simulink library "ncukit"  (R2023b)
settings: Solver=VariableStepAuto  StartTime=0.0  StopTime=10.0  RelTol=1e-3
libraries: simulink x1
settings Model: Creator=sebam  LastModifiedBy=seb
settings SFSimCC: SimUserIncludeDirs=..\lib
settings SFSimCC: SimCustomHeaderCode=|
  | #include <gpio/gpio.h>
  | #include <can/can.h>
settings SFSimCC: SimUserSources=|
  | ..\lib\gpio\gpio.c
  | ..\lib\can\can.c
settings RTWCC: RTWUseSimCustomCode=on  CustomInclude=..\lib
settings RTWCC: CustomHeaderCode=|
  | #include <gpio/gpio.h>
  | #include <can/can.h>
settings RTWCC: CustomSource=|
  | ..\lib\gpio\gpio.c
  | ..\lib\can\can.c

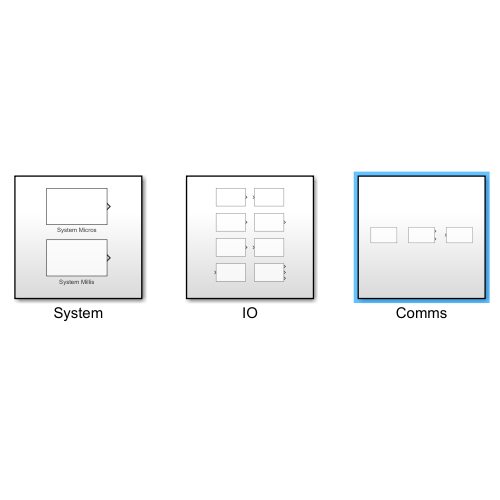
[thumbnail: Simulink's stored preview of the top-level diagram]
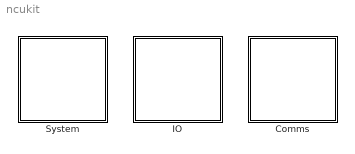
== system ncukit ==
  Comms : Subsystem
  IO : Subsystem
  System : Subsystem

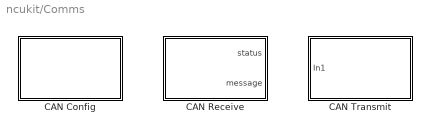
== system ncukit/Comms ==
  CAN Config : Subsystem  mask{bus=can_bus.CAN0, bitrate=can_bitrate.CAN_BITRATE_125K}
      mask Display: image('can_config.png', [25,7,50,50]);
  CAN Receive : Subsystem  mask{bus=can_bus.CAN0}
      mask Display: image('can_receive.png', [25,7,50,50]);
  CAN Transmit : Subsystem  mask{bus=can_bus.CAN0}
      mask Display: image('can_transmit.png', [25,7,50,50]);

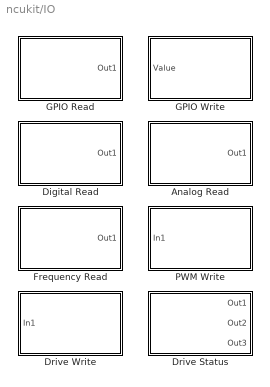
== system ncukit/IO ==
  Analog Read : Subsystem
      mask Display: image('analog_read.png', [25,7,50,50]);
  Digital Read : Subsystem
      mask Display: image('digital_read.png', [25,7,50,50]);
  Drive Status : Subsystem
      mask Display: image('drive_status.png', [25,7,50,50]);
  Drive Write : Subsystem
      mask Display: image('drive_write.png', [25,7,50,50]);
  Frequency Read : Subsystem
      mask Display: image('freq_read.png', [25,7,50,50]);
  GPIO Read : Subsystem  mask{pin=gpio_pin.LED1}
      mask Display: image('gpio_read.png', [25,7,50,50]);
  GPIO Write : Subsystem  mask{pin=gpio_pin.GPIO0}
      mask Display: image('gpio_write.png', [25,7,50,50]);
  PWM Write : Subsystem
      mask Display: image('pwm_write.png', [25,7,50,50]);

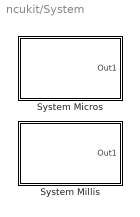
== system ncukit/System ==
  System Micros : Subsystem
      mask Display: image('system_us.png', [25,7,50,50]);
  System Millis : Subsystem
      mask Display: image('system_ms.png', [25,7,50,50]);

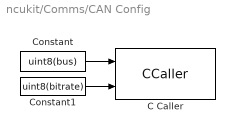
== system ncukit/Comms/CAN Config ==
  C Caller : CCaller  FunctionName=can_set_bitrate  PortSpecificationStruct="%)30     .    V ,   8    (     @         %    \"     (    !     0         %  0 \"0    $    _    07)G3F%M90  4&]R=$YA;64 4V-O<&4     26YD97@     5'EP90      4VEZ90      27-';&]B86P   X    P    !@    @    $          4    (     0    ,    !         !   P!B=7, #@   #     &    \"     0         !0    @    !     P    $         $  # &)U<P .    .     8    (    !          %    \"     $    %     0         0    !0   $EN<'5T    #@   #@    &    \"     8         !0    @    !     0    $         \"0    @               X    X    !@    @    $          4    (     0    4    !         !     %    =6EN=#@    .    ,     8    (    !          %    \"     $    !     0         0  $ ,0    X    P    !@    @    ) @        4    (     0    $    !          (  0      #@   #@    &    \"     0         !0    @    !    !P    $         $     <   !B:71R871E  X    X    !@    @    $          4    (     0    <    !         !     '    8FET<F%T90 .    .     8    (    !          %    \"     $    %     0         0    !0   $EN<'5T    #@   #@    &    \"     8         !0    @    !     0    $         \"0    @           #P/PX   !(    !@    @    $          4    (     0   !,    !         !     3    16YU;3H@8V%N7V)I=')A=&5?=       #@   #     &    \"     0         !0    @    !     0    $         $  ! #$    .    ,     8    (    \"0(        %    \"     $    !     0         \"  $"
  Constant : Constant  Value=uint8(bus)
  Constant1 : Constant  Value=uint8(bitrate)
  wires:
  Constant/1 -> C Caller/1
  Constant1/1 -> C Caller/2

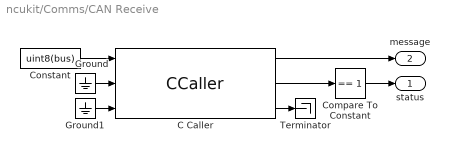
== system ncukit/Comms/CAN Receive ==
  C Caller : CCaller  FunctionName=can_receive  PortSpecificationStruct="%)30     .    . <   8    (     @         %    \"     0    !     0         %  0 \"0    $    _    07)G3F%M90  4&]R=$YA;64 4V-O<&4     26YD97@     5'EP90      4VEZ90      27-';&]B86P   X    P    !@    @    $          4    (     0    ,    !         !   P!O=70 #@   #     &    \"     0         !0    @    !     P    $         $  # &]U=  .    .     8    (    !          %    \"     $    &     0         0   ...(+2112 chars)"
  Compare To Constant : simulink/Logic and Bit Operations/Compare To Constant  relop===  const=1  OutDataTypeStr=boolean
  Constant : Constant  Value=uint8(bus)
  Ground : Ground
  Ground1 : Ground
  Terminator : Terminator
  status : Outport
  message : Outport  Port=2
  wires:
  Ground/1 -> C Caller/2
  Ground1/1 -> C Caller/3
  Constant/1 -> C Caller/1
  C Caller/1 -> message/1
  C Caller/2 -> Compare To Constant/1
  Compare To Constant/1 -> status/1
  C Caller/3 -> Terminator/1

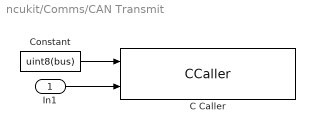
== system ncukit/Comms/CAN Transmit ==
  In1 : Inport
  C Caller : CCaller  FunctionName=can_transmit  PortSpecificationStruct="%)30     .    X ,   8    (     @         %    \"     (    !     0         %  0 \"0    $    _    07)G3F%M90  4&]R=$YA;64 4V-O<&4     26YD97@     5'EP90      4VEZ90      27-';&]B86P   X    P    !@    @    $          4    (     0    ,    !         !   P!B=7, #@   #     &    \"     0         !0    @    !     P    $         $  # &)U<P .    .     8    (    !          %    \"     $    %     0         0    !0   $EN<'5T    #@   #@    &    \"     8         !0    @    !     0    $         \"0    @               X   !     !@    @    $          4    (     0    \\    !         !     /    16YU;3H@8V%N7V)U<U]T  X    P    !@    @    $          4    (     0    $    !         !   0 Q    #@   #     &    \"     D\"        !0    @    !     0    $          @ !       .    .     8    (    !          %    \"     $    '     0         0    !P   &UE<W-A9V4 #@   #@    &    \"     0         !0    @    !    !P    $         $     <   !M97-S86=E  X    X    !@    @    $          4    (     0    4    !         !     %    26YP=70    .    .     8    (    !@         %    \"     $    !     0         )    \"            / _#@   $@    &    \"     0         !0    @    !    %     $         $    !0   !\"=7,Z($-!3E]-15-304=%7T)54P     .    ,     8    (    !          %    \"     $    \"     0         0  ( +3$   X    P    !@    @    ) @        4    (     0    $    !          (  0"
  Constant : Constant  Value=uint8(bus)
  wires:
  In1/1 -> C Caller/2
  Constant/1 -> C Caller/1

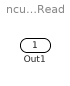
== system ncukit/IO/Analog Read ==
  Out1 : Outport

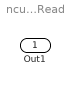
== system ncukit/IO/Digital Read ==
  Out1 : Outport

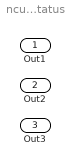
== system ncukit/IO/Drive Status ==
  Out1 : Outport
  Out2 : Outport  Port=2
  Out3 : Outport  Port=3

== system ncukit/IO/Drive Write ==
  In1 : Inport

== system ncukit/IO/Frequency Read ==
  Out1 : Outport

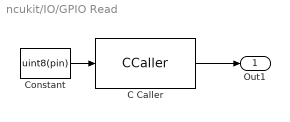
== system ncukit/IO/GPIO Read ==
  C Caller : CCaller  FunctionName=gpio_read  PortSpecificationStruct="%)30     .    N ,   8    (     @         %    \"     (    !     0         %  0 \"0    $    _    07)G3F%M90  4&]R=$YA;64 4V-O<&4     26YD97@     5'EP90      4VEZ90      27-';&]B86P   X    P    !@    @    $          4    (     0    ,    !         !   P!O=70 #@   #     &    \"     0         !0    @    !     P    $         $  # &]U=  .    .     8    (    !          %    \"     $    &     0         0    !@   $]U='!U=   #@   #@    &    \"     8         !0    @    !     0    $         \"0    @               X    X    !@    @    $          4    (     0    <    !         !     '    8F]O;&5A;@ .    ,     8    (    !          %    \"     $    !     0         0  $ ,0    X    P    !@    @    ) @        4    (     0    $    !          (  0      #@   #     &    \"     0         !0    @    !     P    $         $  # '!I;@ .    ,     8    (    !          %    \"     $    #     0         0  , <&EN  X    X    !@    @    $          4    (     0    4    !         !     %    26YP=70    .    .     8    (    !@         %    \"     $    !     0         )    \"               #@   #@    &    \"     0         !0    @    !    !0    $         $     4   !U:6YT.     X    P    !@    @    $          4    (     0    $    !         !   0 Q    #@   #     &    \"     D\"        !0    @    !     0    $          @ !"
  Constant : Constant  Value=uint8(pin)
  Out1 : Outport
  wires:
  Constant/1 -> C Caller/1
  C Caller/1 -> Out1/1

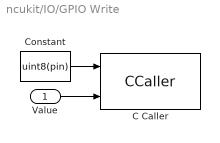
== system ncukit/IO/GPIO Write ==
  Value : Inport
  C Caller : CCaller  FunctionName=gpio_write  PortSpecificationStruct="%)30     .    R ,   8    (     @         %    \"     (    !     0         %  0 \"0    $    _    07)G3F%M90  4&]R=$YA;64 4V-O<&4     26YD97@     5'EP90      4VEZ90      27-';&]B86P   X    P    !@    @    $          4    (     0    ,    !         !   P!P:6X #@   #     &    \"     0         !0    @    !     P    $         $  # '!I;@ .    .     8    (    !          %    \"     $    %     0         0    !0   $EN<'5T    #@   #@    &    \"     8         !0    @    !     0    $         \"0    @               X    X    !@    @    $          4    (     0    4    !         !     %    =6EN=#@    .    ,     8    (    !          %    \"     $    !     0         0  $ ,0    X    P    !@    @    ) @        4    (     0    $    !          (  0      #@   #@    &    \"     0         !0    @    !    !0    $         $     4   !V86QU90    X    X    !@    @    $          4    (     0    4    !         !     %    =F%L=64    .    .     8    (    !          %    \"     $    %     0         0    !0   $EN<'5T    #@   #@    &    \"     8         !0    @    !     0    $         \"0    @           #P/PX    X    !@    @    $          4    (     0    <    !         !     '    8F]O;&5A;@ .    ,     8    (    !          %    \"     $    !     0         0  $ ,0    X    P    !@    @    ) @        4    (     0    $    !          (  0"
  Constant : Constant  Value=uint8(pin)  SampleTime=-1
  wires:
  Constant/1 -> C Caller/1
  Value/1 -> C Caller/2

== system ncukit/IO/PWM Write ==
  In1 : Inport

== system ncukit/System/System Micros ==
  Out1 : Outport

== system ncukit/System/System Millis ==
  Out1 : Outport
